simulink model "Muster_Loesung_Test"  (R2021b)
settings: Solver=FixedStepAuto  StartTime=0.0  StopTime=1  FixedStep=0.001  RelTol=1e-3
values from neighbouring files (symbols this model uses):
  c = 50    [Nils_Bestehorn_WS19_mfile.m]
  d = 0.05    [Nils_Bestehorn_WS19_mfile.m]
  dL = 5*exp(-6)    [Nils_Bestehorn_WS19_mfile.m]
  dM = 1.0*exp(-5)    [Nils_Bestehorn_WS19_mfile.m]
  JL = 2*exp(-5)    [Nils_Bestehorn_WS19_mfile.m]
  JM = 0.125*exp(-5)    [Nils_Bestehorn_WS19_mfile.m]
  LM = 1.0*exp(-3)    [Nils_Bestehorn_WS19_mfile.m]
  ML = 0.25    [Nils_Bestehorn_WS19_mfile.m]
  PHIi = 2.6e-2    (= 0.026)    [Nils_Bestehorn_WS19_mfile.m]
  PHIM = 0.1125    [Nils_Bestehorn_WS19_mfile.m]
  rL = 50*10^(-3)    (= 0.05)    [Nils_Bestehorn_WS19_mfile.m]
  rM = 25*10^(-3)    (= 0.025)    [Nils_Bestehorn_WS19_mfile.m]
  RM = 1.5    [Nils_Bestehorn_WS19_mfile.m]
  Uq = 24    [Nils_Bestehorn_WS19_mfile.m]
settings Model: Creator=nilsb  LastModifiedBy=nilsb

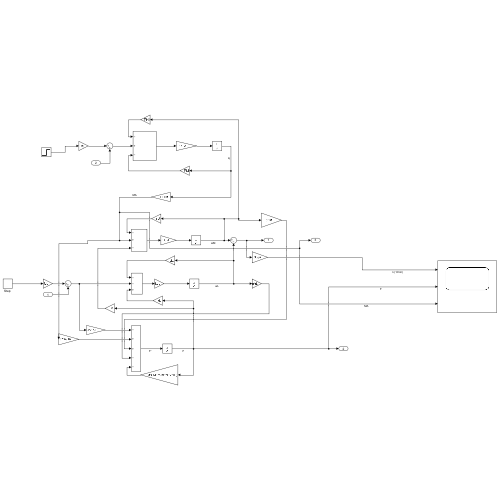
[thumbnail: Simulink's stored preview of the top-level diagram]
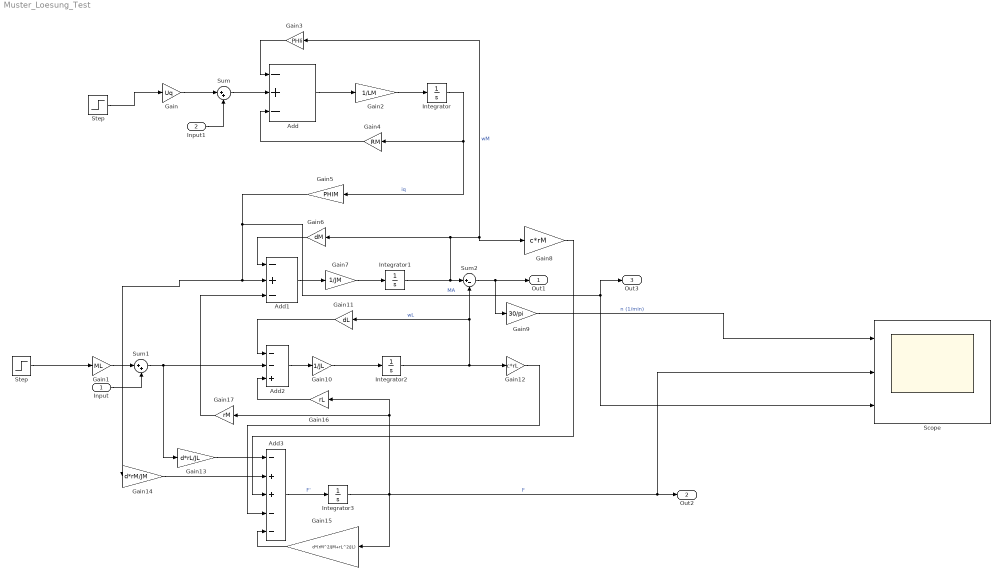
== system Muster_Loesung_Test ==
  Input : Inport
  Input1 : Inport  Port=2
  Add : Sum  Inputs=-+-
  Add1 : Sum  Inputs=-+-
  Add2 : Sum  Inputs=--+
  Add3 : Sum  Inputs=-++--
  Gain : Gain  Gain=Uq
  Gain1 : Gain  Gain=ML
  Gain10 : Gain  Gain=1/JL
  Gain11 : Gain  Gain=dL
  Gain12 : Gain  Gain=c*rL
  Gain13 : Gain  Gain=d*rL/JL
  Gain14 : Gain  Gain=d*rM/JM
  Gain15 : Gain  Gain=d*(rM^2/JM+rL^2/JL)
  Gain16 : Gain  Gain=rL
  Gain17 : Gain  Gain=rM
  Gain2 : Gain  Gain=1/LM
  Gain3 : Gain  Gain=PHIi
  Gain4 : Gain  Gain=RM
  Gain5 : Gain  Gain=PHIM
  Gain6 : Gain  Gain=dM
  Gain7 : Gain  Gain=1/JM
  Gain8 : Gain  Gain=c*rM
  Gain9 : Gain  Gain=30/pi
  Integrator{,1..3} (4 alike) : Integrator
  Scope : Scope  NumInputPorts=3
  Step : Step  Time=0.1  SampleTime=0
  "Step " : Step  Time=0.1  SampleTime=0
  Sum : Sum  Inputs=|++
  Sum1 : Sum  Inputs=|++
  Sum2 : Sum  Inputs=|+-
  Out1 : Outport
  Out2 : Outport  Port=2
  Out3 : Outport  Port=3
  wires:
  Step/1 -> Gain/1
  Gain/1 -> Sum/1
  Sum/1 -> Add/2
  Input1/1 -> Sum/2
  Input/1 -> Sum1/2
  Gain1/1 -> Sum1/1
  Add/1 -> Gain2/1
  Gain3/1 -> Add/1
  Gain2/1 -> Integrator/1
  Integrator/1 -> Gain5/1, Gain4/1  "iq"
  Gain4/1 -> Add/3
  Gain5/1 -> Out3/1, Scope/3, Gain14/1, Add1/2  "MA"
  Gain6/1 -> Add1/1
  Add1/1 -> Gain7/1
  Gain7/1 -> Integrator1/1
  Integrator1/1 -> Gain3/1, Gain8/1, Gain6/1, Sum2/1  "wM"
  Sum2/1 -> Gain9/1, Out1/1
  Gain9/1 -> Scope/1  "n (1/min)"
  Add2/1 -> Gain10/1
  Gain10/1 -> Integrator2/1
  Integrator2/1 -> Gain11/1, Sum2/2, Gain12/1  "wL"
  Gain11/1 -> Add2/1
  Sum1/1 -> Gain13/1, Add2/2
  "Step "/1 -> Gain1/1
  Gain13/1 -> Add3/1
  Gain14/1 -> Add3/2
  Add3/1 -> Integrator3/1  "F'"
  Integrator3/1 -> Out2/1, Scope/2, Gain15/1, Gain17/1, Gain16/1  "F"
  Gain15/1 -> Add3/5
  Gain16/1 -> Add2/3
  Gain17/1 -> Add1/3
  Gain8/1 -> Add3/3
  Gain12/1 -> Add3/4
